simulink model "manning_3test_linear"  (R2022b)
settings: Solver=VariableStepAuto  StartTime=0.0  StopTime=5*34416  RelTol=1e-3
undefined symbols (not defined in the file): gain, yd_ds
settings Model: Creator=chuan  LastModifiedBy=chuan

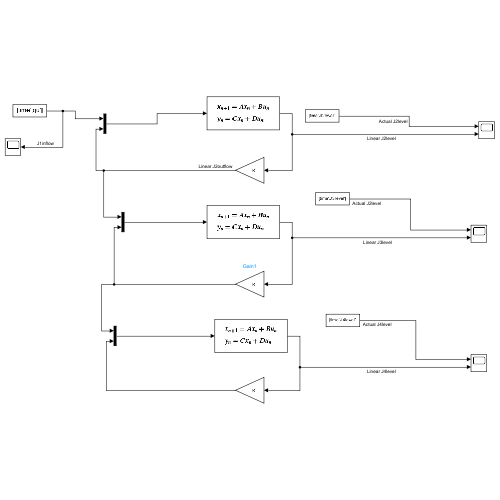
[thumbnail: Simulink's stored preview of the top-level diagram]
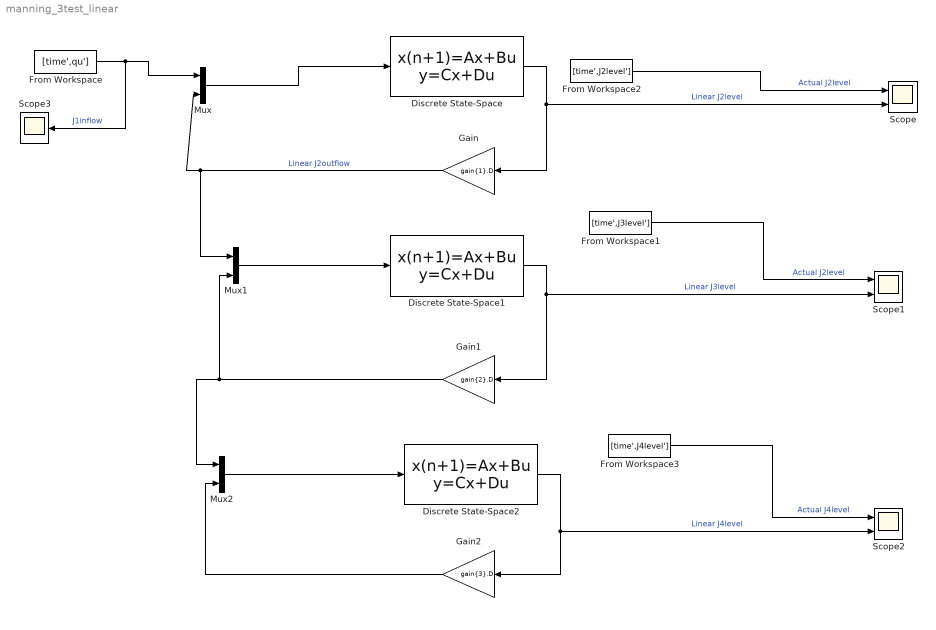
== system manning_3test_linear ==
  Discrete State-Space : DiscreteStateSpace  A=yd_ds{1}.A  B=yd_ds{1}.B  C=yd_ds{1}.C  D=yd_ds{1}.D  SampleTime=yd_ds{1}.Ts
  Discrete State-Space1 : DiscreteStateSpace  A=yd_ds{2}.A  B=yd_ds{2}.B  C=yd_ds{2}.C  D=yd_ds{2}.D  SampleTime=yd_ds{2}.Ts
  Discrete State-Space2 : DiscreteStateSpace  A=yd_ds{3}.A  B=yd_ds{3}.B  C=yd_ds{3}.C  D=yd_ds{3}.D  SampleTime=yd_ds{3}.Ts
  From Workspace : FromWorkspace  VariableName=[time',qu']
  From Workspace1 : FromWorkspace  VariableName=[time',J3level']
  From Workspace2 : FromWorkspace  VariableName=[time',J2level']
  From Workspace3 : FromWorkspace  VariableName=[time',J4level']
  Gain : Gain  Gain=gain{1}.D
  Gain1 : Gain  Gain=gain{2}.D
  Gain2 : Gain  Gain=gain{3}.D
  Mux : Mux  Inputs=2
  Mux1 : Mux  Inputs=2
  Mux2 : Mux  Inputs=2
  Scope : Scope  NumInputPorts=2
  Scope1 : Scope  NumInputPorts=2
  Scope2 : Scope  NumInputPorts=2
  Scope3 : Scope
  wires:
  Discrete State-Space/1 -> Gain/1, Scope/2  "Linear J2level"
  Gain/1 -> Mux1/1, Mux/2  "Linear J2outflow"
  Mux/1 -> Discrete State-Space/1
  From Workspace/1 -> Scope3/1, Mux/1  "J1inflow"
  From Workspace2/1 -> Scope/1  "Actual J2level"
  Gain1/1 -> Mux2/1, Mux1/2
  Mux1/1 -> Discrete State-Space1/1
  Discrete State-Space1/1 -> Gain1/1, Scope1/2  "Linear J3level"
  From Workspace1/1 -> Scope1/1  "Actual J2level"
  Mux2/1 -> Discrete State-Space2/1
  Discrete State-Space2/1 -> Gain2/1, Scope2/2  "Linear J4level"
  Gain2/1 -> Mux2/2
  From Workspace3/1 -> Scope2/1  "Actual J4level"
